simulink model "Drdo_sim_2"  (R2021a)
settings: Solver=VariableStepAuto  StartTime=0.0  StopTime=200  RelTol=1e-3
undefined symbols (not defined in the file): Ion, Lithium
libraries: spsDiodeLib x8, spsMosfetLib x8, spsBatteryLib x3, spsCurrentMeasurementLib x2, simulink x2, spsParallelRLCBranchLib x2, spsVoltageMeasurementLib x2, spsIdealSwitchLib x1, spspowerguiLib x1
settings Model: Creator=rachi  LastModifiedBy=rachi
settings SolverCC: ZeroCrossAlgorithm=Adaptive
settings DebuggingCC: IgnoredZcDiagnostic=none

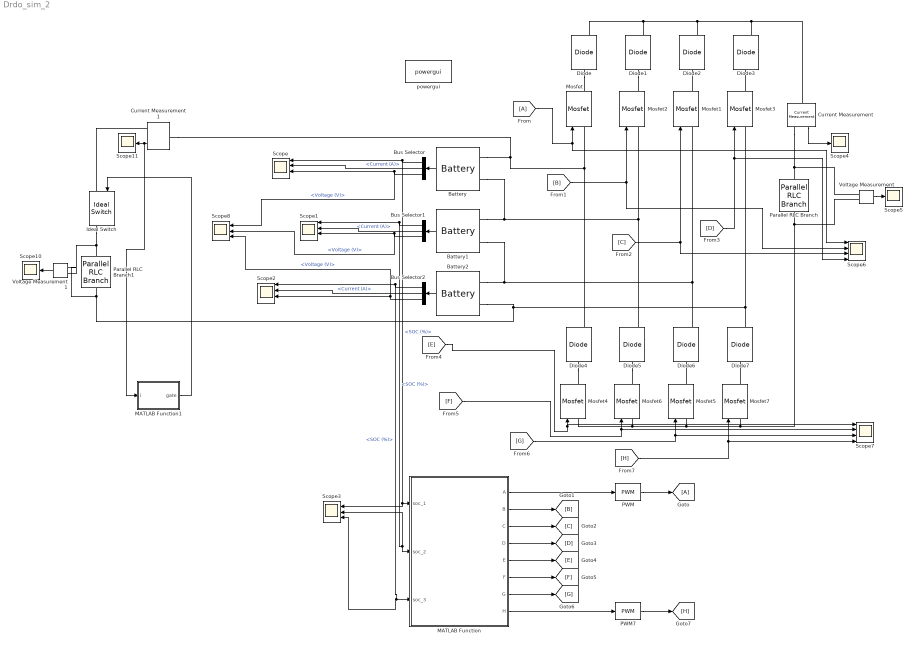
== system Drdo_sim_2 ==
  Battery : spsBatteryLib/Battery  BatType=Lithium-Ion  ShowTempParam=off  ThermalPreset=no  ShowAgeParam=off  NomV=3.6  NomQ=7.5  SOC=57.5  Batt_Tr=30  PresetModel=on  MaxQ=7.5  MinV=2.7  FullV=4.1904  Dis_rate=3.2609  R=0.0048  Normal_OP=6.7826  expZone="[3.8894     0.36848]"  current=[6.5 13 32.5]  Units=Time  Tci=20  NomT=20  T2=-30  MaxQ2=4.8  FullV2=7.1  Normal_OP2=5.655  expZone2="[6.58           1]"  Rca=0.6  ti=2000  Dp=0  Neq0=0  Tsim=1e6  Ta1=25  Qeol=5.4*0.9  Reol=0.013333*1.2  Char_age=[2.3478, 3]  Dis_age=[2.3478, 10]  N1=1500  N2=10500  N3=1000  N4=1400  Ta2=45  N5=950
  Battery1 : spsBatteryLib/Battery  BatType=Lithium-Ion  ShowTempParam=off  ThermalPreset=no  ShowAgeParam=off  NomV=3.6  NomQ=7.5  SOC=57.7  Batt_Tr=30  PresetModel=on  MaxQ=7.5  MinV=2.7  FullV=4.1904  Dis_rate=3.2609  R=0.0048  Normal_OP=6.7826  expZone="[3.8894     0.36848]"  current=[6.5 13 32.5]  Units=Time  Tci=20  NomT=20  T2=-30  MaxQ2=4.8  FullV2=7.1  Normal_OP2=5.655  expZone2="[6.58           1]"  Rca=0.6  ti=2000  Dp=0  Neq0=0  Tsim=1e6  Ta1=25  Qeol=5.4*0.9  Reol=0.013333*1.2  Char_age=[2.3478, 3]  Dis_age=[2.3478, 10]  N1=1500  N2=10500  N3=1000  N4=1400  Ta2=45  N5=950
  Battery2 : spsBatteryLib/Battery  BatType=Lithium-Ion  ShowTempParam=off  ThermalPreset=no  ShowAgeParam=off  NomV=3.6  NomQ=7.5  SOC=57.6  Batt_Tr=30  PresetModel=on  MaxQ=7.5  MinV=2.7  FullV=4.1904  Dis_rate=3.2609  R=0.0048  Normal_OP=6.7826  expZone="[3.8894     0.36848]"  current=[6.5 13 32.5]  Units=Time  Tci=20  NomT=20  T2=-30  MaxQ2=4.8  FullV2=7.1  Normal_OP2=5.655  expZone2="[6.58           1]"  Rca=0.6  ti=2000  Dp=0  Neq0=0  Tsim=1e6  Ta1=25  Qeol=5.4*0.9  Reol=0.013333*1.2  Char_age=[2.3478, 3]  Dis_age=[2.3478, 10]  N1=1500  N2=10500  N3=1000  N4=1400  Ta2=45  N5=950
  Bus Selector : BusSelector  OutputSignals=SOC (%),Current (A),Voltage (V)
  Bus Selector1 : BusSelector  OutputSignals=SOC (%),Current (A),Voltage (V)
  Bus Selector2 : BusSelector  OutputSignals=SOC (%),Current (A),Voltage (V)
  Current Measurement : spsCurrentMeasurementLib/Current Measurement  PhasorSimulation=off  OutputType=Complex  PSBequivalent=0
  Current Measurement1 : spsCurrentMeasurementLib/Current Measurement  PhasorSimulation=off  OutputType=Complex  PSBequivalent=0
  Diode{,1..7} (8 alike) : spsDiodeLib/Diode  Ron=0.001  Lon=0  Vf=0.8  IC=0  UseSnubber=0  Rs=500  Cs=250e-9  Measurements=on
  Ideal Switch : spsIdealSwitchLib/Ideal Switch  Ron=0.001  Lon=0  IC=0  Rs=1e5  Cs=inf  Measurements=on
  MATLAB Function : MATLAB Function  TreatAsAtomicUnit=on
  MATLAB Function1 : MATLAB Function  TreatAsAtomicUnit=on
  Mosfet{,1..7} (8 alike) : spsMosfetLib/Mosfet  Ron=0.1  Lon=0  Rd=0.01  Vfd=0  IC=0  Rs=1e5  Cs=inf  Measurements=on
  PWM : simulink/Discontinuities/PWM  DisableCoverage=on  Period=0.004  DisallowZeroDutyCycle=off  RunAtFixedTimeIntervals=off  SampleTime=0.1
  PWM7 : simulink/Discontinuities/PWM  DisableCoverage=on  Period=0.004  DisallowZeroDutyCycle=off  RunAtFixedTimeIntervals=off  SampleTime=0.1
  Parallel RLC Branch : spsParallelRLCBranchLib/Parallel RLC Branch  LConnTagsString=a  RConnTagsString=__new0  BranchType=L  Resistance=1  Inductance=5e-3  SetiL0=off  InitialCurrent=0  Capacitance=1e-6  Setx0=off  InitialVoltage=0  Measurements=None
  Parallel RLC Branch1 : spsParallelRLCBranchLib/Parallel RLC Branch  LConnTagsString=a  RConnTagsString=__new0  BranchType=R  Resistance=10  Inductance=1e-3  SetiL0=off  InitialCurrent=0  Capacitance=1e-6  Setx0=off  InitialVoltage=0  Measurements=None
  Scope{,1..2,6..7} (5 alike) : Scope  NumInputPorts=4
  Scope{4..5,10..11} (4 alike) : Scope
  Scope3 : Scope  NumInputPorts=3
  Scope8 : Scope  NumInputPorts=3
  Voltage Measurement : spsVoltageMeasurementLib/Voltage Measurement  PhasorSimulation=off  OutputType=Complex  PSBequivalent=0
  Voltage Measurement1 : spsVoltageMeasurementLib/Voltage Measurement  PhasorSimulation=off  OutputType=Complex  PSBequivalent=0
  powergui : spspowerguiLib/powergui  Priority=1  SimulationMode=Continuous  SampleTime=50e-6  frequency=60  Iterations=50  frequencyindice=0  Pbase=100e6  ErrMax=1e-4  UnitsV=kV  UnitsW=MW  buscounter=0  FunctionMessages=off  echomessages=off  EnableUseOfTLC=off  CurrentSourceSwitches=off  DisableSnubberDevices=off  DisableRonSwitches=off  DisableVfSwitches=off  DisplayEquations=off  AutomaticDiscreteSolvers=off  SolverType=Tustin/Backward Euler (TBE)  Interpol=off  ExternalGateDelay=off  methode=off  Ts=100  x0status=blocks  SPID=on  SwTol=0  HookPort=off  NonlinearTolerance=1e-4  nMaxIteration=100  ContinueOnMaxIteration=off  RestoreLinks=warning  ResistiveCurrentMeasurement=off  Frange=[0:2:500]  Ylog=off  Xlog=on  ShowGrid=off  save=off  variable=ZData  structure=0  ZoomFFT=off  StartTime=0.0  cycles=1  DisplayStyle=1  fundamental=60  FreqAxis=off  MaxFrequency=1000  frequencyindicesteady=1  RmsSteady=1  display=off
  wires:
  Battery/1 -> Bus Selector/1
  Battery1/1 -> Bus Selector1/1
  Battery2/1 -> Bus Selector2/1
  Bus Selector/1 -> Scope3/1, MATLAB Function/1(soc_1), Scope/1  "<SOC (%)>"
  Bus Selector/2 -> Scope/2  "<Current (A)>"
  Bus Selector/3 -> Scope8/1, Scope/3  "<Voltage (V)>"
  Bus Selector1/2 -> Scope1/2  "<Current (A)>"
  Bus Selector1/3 -> Scope8/2, Scope1/3  "<Voltage (V)>"
  Bus Selector1/1 -> Scope3/2, MATLAB Function/2(soc_2), Scope1/1  "<SOC (%)>"
  Bus Selector2/2 -> Scope2/2  "<Current (A)>"
  Bus Selector2/3 -> Scope8/3, Scope2/3  "<Voltage (V)>"
  Bus Selector2/1 -> Scope3/3, MATLAB Function/3(soc_3), Scope2/1  "<SOC (%)>"
  MATLAB Function/2(B) -> [B]
  MATLAB Function/3(C) -> [C]
  MATLAB Function/4(D) -> [D]
  MATLAB Function/5(E) -> [E]
  MATLAB Function/6(F) -> [F]
  MATLAB Function/7(G) -> [G]
  MATLAB Function/8(H) -> PWM7/1
  [A] -> Mosfet/1, Scope6/1
  [B] -> Scope6/2, Mosfet2/1
  [C] -> Mosfet1/1, Scope6/3
  [D] -> Scope6/4, Mosfet3/1
  [E] -> Scope7/1, Mosfet4/1
  [F] -> Scope7/2, Mosfet6/1
  [G] -> Scope7/3, Mosfet5/1
  [H] -> Scope7/4, Mosfet7/1
  Current Measurement/1 -> Scope4/1
  Voltage Measurement/1 -> Scope5/1
  MATLAB Function/1(A) -> PWM/1
  PWM/1 -> [A]
  PWM7/1 -> [H]
  Current Measurement1/1 -> MATLAB Function1/1(i), Scope11/1
  Voltage Measurement1/1 -> Scope10/1
  MATLAB Function1/1(gate) -> Ideal Switch/1
  connections:
  Battery/LConn1 -- Mosfet/LConn1 -- Diode4/RConn1 -- Current Measurement1/LConn1
  Battery1/LConn1 -- Battery/LConn2 -- Diode5/RConn1 -- Mosfet2/LConn1
  Battery2/LConn1 -- Mosfet1/LConn1 -- Diode6/RConn1 -- Battery1/LConn2
  Battery2/LConn2 -- Voltage Measurement1/LConn2 -- Parallel RLC Branch1/RConn1 -- Mosfet3/LConn1 -- Diode7/RConn1
  Diode/LConn1 -- Mosfet/RConn1
  Diode1/LConn1 -- Mosfet2/RConn1
  Mosfet1/RConn1 -- Diode2/LConn1
  Mosfet3/RConn1 -- Diode3/LConn1
  Diode4/LConn1 -- Mosfet4/RConn1
  Diode5/LConn1 -- Mosfet6/RConn1
  Mosfet5/RConn1 -- Diode6/LConn1
  Mosfet7/RConn1 -- Diode7/LConn1
  Diode/RConn1 -- Diode1/RConn1 -- Diode2/RConn1 -- Current Measurement/LConn1 -- Diode3/RConn1
  Mosfet7/LConn1 -- Voltage Measurement/LConn2 -- Parallel RLC Branch/LConn1 -- Mosfet4/LConn1 -- Mosfet6/LConn1 -- Mosfet5/LConn1
  Current Measurement/RConn1 -- Voltage Measurement/LConn1 -- Parallel RLC Branch/RConn1
  Ideal Switch/RConn1 -- Voltage Measurement1/LConn1 -- Parallel RLC Branch1/LConn1
  Current Measurement1/RConn1 -- Ideal Switch/LConn1

== matlab function Drdo_sim_2/MATLAB Function1 ==
  data: i input; gate output
function gate = fcn(i)
gate=0;
if i>3
    gate=0;
end

== matlab function Drdo_sim_2/MATLAB Function ==
  data: soc_1 input; A output; soc_2 input; soc_3 input; B output; C output; D output; E output; F output; G output; H output
function [A,B,C,D,E,F,G,H]= fcn(soc_1, soc_2, soc_3)
A=0;
B=0;
C=0;
D=0;
E=0;
F=0;
G=0;
H=0;
soc1=round(soc_1 * 10000)/10000;
soc2=round(soc_2 * 10000)/10000;
soc3=round(soc_3 * 10000)/10000;
duty_cycle=0.30;
if soc1 == soc2 && soc2 == soc3
    %do nothing
else  
    if soc1>=soc2
        if soc2>=soc3 %soc3 is smallest
            G=1;
            D=1;
            A=duty_cycle;
            H=duty_cycle;
        else %soc2 is smallest
            F=1;
            C=1;
            A=duty_cycle;
            H=duty_cycle;
        end
    elseif soc1>=soc3 %soc3 is smallest
        G=1;
        D=1;
        A=duty_cycle;
        H=duty_cycle;
    elseif soc3>=soc1 %soc1 is smallest
        E=1;
        B=1;
        A=duty_cycle;
        H=duty_cycle;
    end
end
